simulink model "simulation_regulation"  (Simulink 7.7)
settings: Solver=ode45  StartTime=0.999  StopTime=1.007  RelTol=1e-3
values from neighbouring files (symbols this model uses):
  bruit_bf = 0    [Vout18V.m]
  pertu_sortie_bf = 1    [Vout18V.m]
undefined symbols (not defined in the file or in its folder): Rd_tf
libraries: cstblocks x4
settings Model: Creator=adminportog  LastModifiedBy=Nicolas
settings OptimizationCC: InitFltsAndDblsToZero=on
settings DebuggingCC: StrictBusMsg=Warning

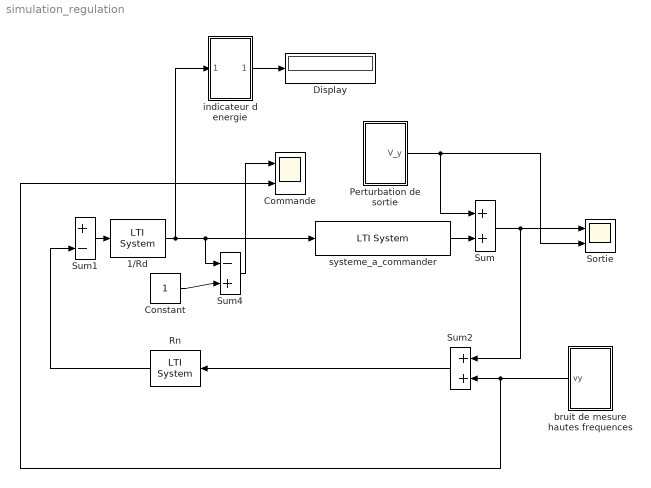
== system simulation_regulation ==
  1/Rd : cstblocks/LTI System  SystemSampleTime=-1  sys=1/Rd_tf  IC=[]
  Commande : Scope  NumInputPorts=2
      settings: TickLabels=on  TimeRange=10  YMin=-0.0006~-0.125  YMax=0.001~0.125  MaxDataPoints=50000
  Constant : Constant
  Display : Display
  Perturbation de sortie : Subsystem
  Rn : cstblocks/LTI System  SystemSampleTime=-1  sys=Rn_tf  IC=[]
  Sortie : Scope  NumInputPorts=2
      settings: TickLabels=on  TimeRange=10  YMin=-5~-5  YMax=5~5  MaxDataPoints=50000
  Sum : Sum
  Sum1 : Sum  Inputs=|+-
  Sum2 : Sum
  Sum4 : Sum  Inputs=|-+
  bruit de mesure hautes frequences : Subsystem
  indicateur d energie : Subsystem
  systeme_a_commander : cstblocks/LTI System  SystemSampleTime=-1  sys=G_nominal_commande  IC=[]
  wires:
  systeme_a_commander/1 -> Sum/2
  Sum/1 -> Sortie/1, Sum2/1
  Sum1/1 -> 1/Rd/1
  1/Rd/1 -> indicateur d energie/1(In1), systeme_a_commander/1, Sum4/1
  Sum2/1 -> Rn/1
  bruit de mesure hautes frequences/1(vy) -> Sum2/2, Commande/2
  Perturbation de sortie/1(V_y) -> Sum/1, Sortie/2
  indicateur d energie/1(Out1) -> Display/1
  Rn/1 -> Sum1/2
  Constant/1 -> Sum4/2
  Sum4/1 -> Commande/1

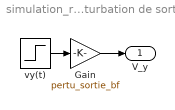
== system simulation_regulation/Perturbation de sortie ==
  Gain : Gain  Gain=pertu_sortie_bf
  vy(t) : Step  SampleTime=0
  V_y : Outport
  wires:
  vy(t)/1 -> Gain/1
  Gain/1 -> V_y/1

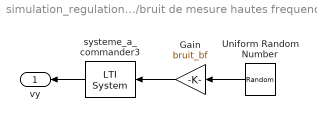
== system simulation_regulation/bruit de mesure hautes frequences ==
  Gain : Gain  Gain=bruit_bf
  Uniform Random Number : UniformRandomNumber  Minimum=-0.1  Maximum=0.1  SampleTime=0
  systeme_a_commander3 : cstblocks/LTI System  SystemSampleTime=-1  sys=tf([1 8*1e4],[1 1e5])  IC=[]
  vy : Outport
  wires:
  Uniform Random Number/1 -> Gain/1
  systeme_a_commander3/1 -> vy/1
  Gain/1 -> systeme_a_commander3/1

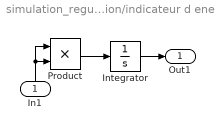
== system simulation_regulation/indicateur d energie ==
  In1 : Inport
  Integrator : Integrator
  Product : Product  RndMeth=Zero
  Out1 : Outport
  wires:
  Product/1 -> Integrator/1
  In1/1 -> Product/2, Product/1
  Integrator/1 -> Out1/1
